simulink model "ADRC"  (R2018a)
settings: Solver=VariableStepAuto  StartTime=0.0  StopTime=10.0  RelTol=1e-3
settings Model: Creator=R-YDL  LastModifiedBy=R-YDL

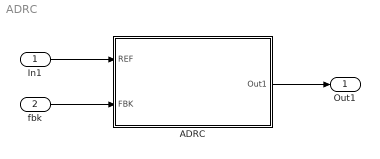
== system ADRC ==
  In1 : Inport
  fbk : Inport  Port=2
  ADRC : Subsystem  mask{alpha0=0, delta0=0, r0=0, alpha1=0, delta1=0, beta1=0, beta2=0, alpha2=0, delta2=0, b0=0, k=0}
      mask prompts: alpha0 "跟踪因子α"; delta0 "滤波因子δ"; r0 "速度因子r0"; alpha1 "跟踪因子α"; delta1 "滤波因子δ"; beta1 "校正增益β1"; beta2 "校正增益β2"; alpha2 "跟踪因子α"; delta2 "滤波因子δ"; b0 "补偿因子b0"; k "调节增益k"
      mask DialogControl Container3 Prompt: TD
      mask DialogControl Container4 Prompt: ESO
      mask DialogControl Container5 Prompt: NLSEF
  Out1 : Outport
  wires:
  In1/1 -> ADRC/1(REF)
  fbk/1 -> ADRC/2(FBK)
  ADRC/1(Out1) -> Out1/1

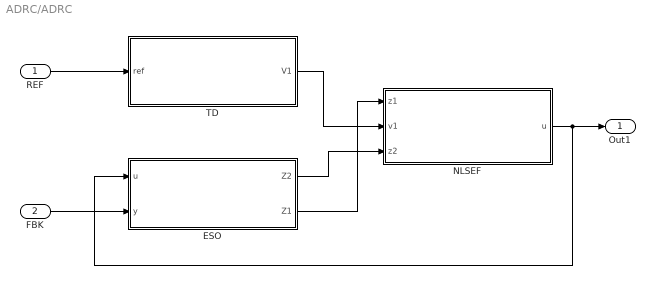
== system ADRC/ADRC ==
  REF : Inport
  FBK : Inport  Port=2
  "ESO " : Subsystem
  NLSEF : Subsystem
  TD : Subsystem
  Out1 : Outport
  wires:
  NLSEF/1(u) -> "ESO "/1(u), Out1/1
  TD/1(V1) -> NLSEF/2(v1)
  REF/1 -> TD/1(ref)
  "ESO "/2(Z1) -> NLSEF/1(z1)
  "ESO "/1(Z2) -> NLSEF/3(z2)
  FBK/1 -> "ESO "/2(y)

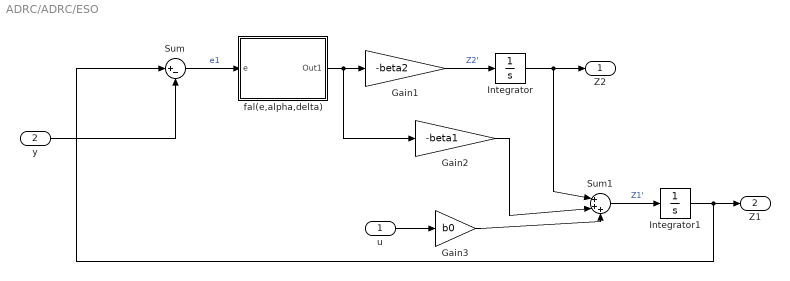
== system ADRC/ADRC/ESO  ==
  u : Inport
  y : Inport  Port=2
  Gain1 : Gain  Gain=-beta2
  Gain2 : Gain  Gain=-beta1
  Gain3 : Gain  Gain=b0
  Integrator : Integrator
  Integrator1 : Integrator
  Sum : Sum  Inputs=|+-
  Sum1 : Sum  Inputs=|+++
  fal(e,alpha,delta) : Subsystem  mask{alpha=alpha1, delta=delta1}
      mask prompts: alpha "跟踪因子α"; delta "滤波因子δ"
  Z2 : Outport
  Z1 : Outport  Port=2
  wires:
  Sum/1 -> fal(e,alpha,delta)/1(e)  "e1"
  Gain1/1 -> Integrator/1  "Z2'"
  Integrator/1 -> Sum1/1, Z2/1
  Sum1/1 -> Integrator1/1  "Z1'"
  Integrator1/1 -> Sum/1, Z1/1
  fal(e,alpha,delta)/1(Out1) -> Gain2/1, Gain1/1
  u/1 -> Gain3/1
  Gain3/1 -> Sum1/3
  Gain2/1 -> Sum1/2
  y/1 -> Sum/2

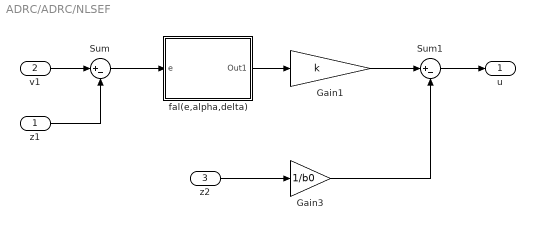
== system ADRC/ADRC/NLSEF ==
  z1 : Inport
  v1 : Inport  Port=2
  z2 : Inport  Port=3
  Gain1 : Gain  Gain=k
  Gain3 : Gain  Gain=1/b0
  Sum : Sum  Inputs=|+-
  Sum1 : Sum  Inputs=|+-
  fal(e,alpha,delta) : Subsystem  mask{alpha=alpha2, delta=delta2}
      mask prompts: alpha "跟踪因子α"; delta "滤波因子δ"
  u : Outport
  wires:
  Sum/1 -> fal(e,alpha,delta)/1(e)
  fal(e,alpha,delta)/1(Out1) -> Gain1/1
  z1/1 -> Sum/2
  v1/1 -> Sum/1
  z2/1 -> Gain3/1
  Sum1/1 -> u/1
  Gain1/1 -> Sum1/1
  Gain3/1 -> Sum1/2

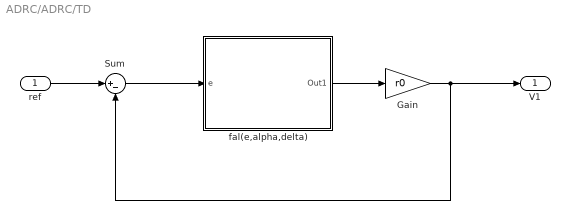
== system ADRC/ADRC/TD ==
  ref : Inport
  Gain : Gain  Gain=r0
  Sum : Sum  Inputs=|+-
  fal(e,alpha,delta) : Subsystem  mask{alpha=alpha0, delta=delta0}
      mask prompts: alpha "跟踪因子α"; delta "滤波因子δ"
  V1 : Outport
  wires:
  Gain/1 -> V1/1, Sum/2
  ref/1 -> Sum/1
  fal(e,alpha,delta)/1(Out1) -> Gain/1
  Sum/1 -> fal(e,alpha,delta)/1(e)

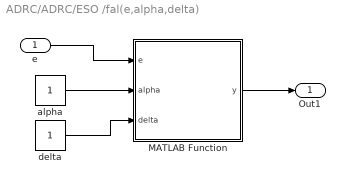
== system ADRC/ADRC/ESO /fal(e,alpha,delta) ==
  e : Inport
  MATLAB Function : MATLAB Function  TreatAsAtomicUnit=on  mask{alpha=0, delta=0}
      mask prompts: alpha "跟踪因子"; delta "滤波因子"
  alpha : Constant
  delta : Constant
  Out1 : Outport
  wires:
  MATLAB Function/1(y) -> Out1/1
  alpha/1 -> MATLAB Function/2(alpha)
  delta/1 -> MATLAB Function/3(delta)
  e/1 -> MATLAB Function/1(e)

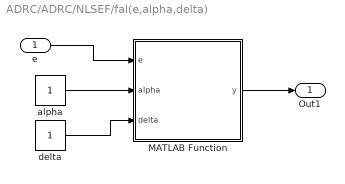
== system ADRC/ADRC/NLSEF/fal(e,alpha,delta) ==
  e : Inport
  MATLAB Function : MATLAB Function  TreatAsAtomicUnit=on  mask{alpha=0, delta=0}
      mask prompts: alpha "跟踪因子"; delta "滤波因子"
  alpha : Constant
  delta : Constant
  Out1 : Outport
  wires:
  MATLAB Function/1(y) -> Out1/1
  alpha/1 -> MATLAB Function/2(alpha)
  delta/1 -> MATLAB Function/3(delta)
  e/1 -> MATLAB Function/1(e)

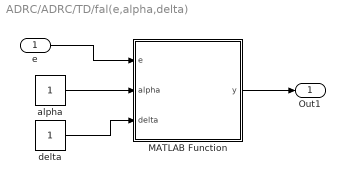
== system ADRC/ADRC/TD/fal(e,alpha,delta) ==
  e : Inport
  MATLAB Function : MATLAB Function  TreatAsAtomicUnit=on  mask{alpha=0, delta=0}
      mask prompts: alpha "跟踪因子"; delta "滤波因子"
  alpha : Constant
  delta : Constant
  Out1 : Outport
  wires:
  MATLAB Function/1(y) -> Out1/1
  alpha/1 -> MATLAB Function/2(alpha)
  delta/1 -> MATLAB Function/3(delta)
  e/1 -> MATLAB Function/1(e)

== matlab function ADRC/ESO /fal(e,alpha,delta)/MATLAB Function ==
  data: e input; y output; alpha input; delta input
function y = fcn(e,alpha,delta)

if abs(e)>delta
    y = (abs(e))^alpha * sign(e);
else
    y = e/(delta^(1 - alpha));
end

end

== matlab function ADRC/TD/fal(e,alpha,delta)/MATLAB Function ==
  data: e input; y output; alpha input; delta input
function y = fcn(e,alpha,delta)

if abs(e)>delta
    y = (abs(e))^alpha * sign(e);
else
    y = e/(delta^(1 - alpha));
end

end

== matlab function ADRC/NLSEF/fal(e,alpha,delta)/MATLAB Function ==
  data: e input; y output; alpha input; delta input
function y = fcn(e,alpha,delta)

if abs(e)>delta
    y = (abs(e))^alpha * sign(e);
else
    y = e/(delta^(1 - alpha));
end

end
